simulink model "testBuffer"  (R2015a)
settings: Solver=ode3  StartTime=0.0  StopTime=10.0  FixedStep=0.016  RelTol=1e-3
libraries: simulink x1
settings Model: Creator=go  LastModifiedBy=go

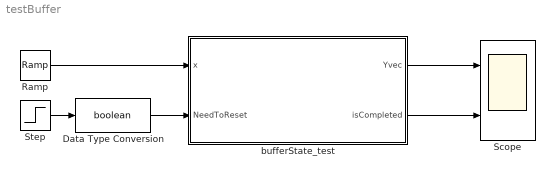
== system testBuffer ==
  Data Type Conversion : DataTypeConversion  OutDataTypeStr=boolean
  Ramp : simulink/Sources/Ramp  slope=1  start=0  X0=0
  Scope : Scope  NumInputPorts=2
      settings: YMin=-5~-5  YMax=5~5
  Step : Step  Time=0.5  Before=1  After=0  SampleTime=0
  bufferState_test : MATLAB Function  TreatAsAtomicUnit=on
  wires:
  Ramp/1 -> bufferState_test/1(x)
  Data Type Conversion/1 -> bufferState_test/2(NeedToReset)
  bufferState_test/1(Yvec) -> Scope/1
  bufferState_test/2(isCompleted) -> Scope/2
  Step/1 -> Data Type Conversion/1

== matlab function testBuffer/bufferState_test ==
  data: x input; Yvec output; NeedToReset input; isCompleted output
function [Yvec,isCompleted] = bufferState( x, NeedToReset)
%  Summary of this function goes here
%  Detailed explanation goes here

 persistent xbuffer;
 persistent cont;
 
 BuffTimeMax = 3; %[sec]
 dt = 0.016;      %[sec]
 idxBufferMax = round(BuffTimeMax / dt);

 if ( isempty(xbuffer) || isempty(cont) )
     xbuffer = zeros(1,idxBufferMax);
     cont = 0;
 end
 
 if ( NeedToReset == true )     
     isCompleted = false;
     xbuffer = zeros(1,idxBufferMax);
     xbufferTemp = xbuffer(2:idxBufferMax);
     cont = 0;
 else
     xbufferTemp = xbuffer(2:idxBufferMax);
     xbuffer = [xbufferTemp x];
           
     if ( cont >= idxBufferMax)
          cont = idxBufferMax;    
          isCompleted = true;
     else
          isCompleted = false;
          cont = cont + 1  ;
     end
 end
 
 Yvec = xbuffer;
 
end
